simulink model "caso_non_noto_scalare"  (R2024b)
settings: Solver=VariableStepAuto  StartTime=0.0  StopTime=10.0  RelTol=1e-3
settings Model: Creator=david  LastModifiedBy=david

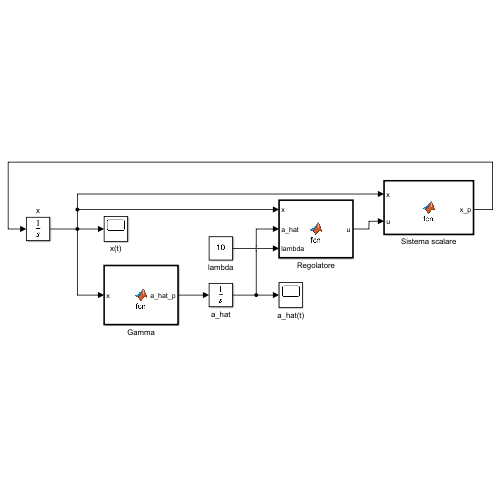
[thumbnail: Simulink's stored preview of the top-level diagram]
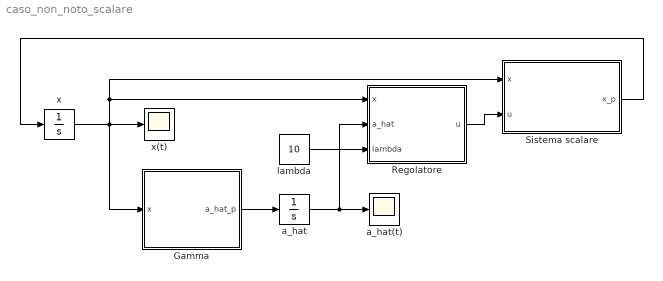
== system caso_non_noto_scalare ==
  Gamma : MATLAB Function  TreatAsAtomicUnit=on
  Regolatore : MATLAB Function  TreatAsAtomicUnit=on
  Sistema scalare : MATLAB Function  TreatAsAtomicUnit=on
  a_hat : Integrator  InitialCondition=14
  a_hat(t) : Scope
  lambda : Constant  Value=10  VectorParams1D=off
  x : Integrator  InitialCondition=1
  x(t) : Scope
  wires:
  x/1 -> Sistema scalare/1(x), Regolatore/1(x), x(t)/1, Gamma/1(x)
  Regolatore/1(u) -> Sistema scalare/2(u)
  Gamma/1(a_hat_p) -> a_hat/1
  Sistema scalare/1(x_p) -> x/1
  lambda/1 -> Regolatore/3(lambda)
  a_hat/1 -> Regolatore/2(a_hat), a_hat(t)/1

== matlab function caso_non_noto_scalare/Sistema scalare ==
  data: x input; x_p output; u input
function x_p = fcn(x,u)

a=10;
x_p = a*x + u;

== matlab function caso_non_noto_scalare/Gamma ==
  data: x input; a_hat_p output
function a_hat_p = fcn(x)

a_hat_p = x^2; %stima dell'errore

== matlab function caso_non_noto_scalare/Regolatore ==
  data: x input; u output; a_hat input; lambda input
function u = fcn(x,a_hat,lambda)

u = -a_hat*x -lambda*x;
